simulink model "playback_data"  (R2015a)
settings: Solver=FixedStepDiscrete  SolverMode=SingleTasking  StartTime=76  StopTime=110  FixedStep=sample_time  RelTol=1e-3
undefined symbols (not defined in the file): A1_notch_f1, A2_notch_f1, A_kalman_swing_load, A_kalman_transverse, A_kalman_vertical, A_lpf_accelerometer, A_lpf_dtau, A_lpf_fourbar_angles, A_lpf_imu, A_lpf_lateral_angle, B1_lpf_accelerometer, B1_lpf_dtau, B1_lpf_fourbar_angles, B1_lpf_imu, B1_lpf_lateral_angle, B1_notch_f1, B2_lpf_accelerometer, B2_lpf_dtau, B2_lpf_fourbar_angles, B2_lpf_imu, B2_lpf_lateral_angle, B2_notch_f1, B_dx_versus_x0, B_kalman_swing_load, B_kalman_transverse, B_kalman_vertical, backwards_K_sag_of_t, backwards_P_sag_of_t, C_kalman_swing_load, C_kalman_transverse, C_kalman_vertical, com_leg_motor, com_torso, contact_threshold, control_start_time, d_ankle_to_foot, d_vertical_com, desired_com_forward_velocity, desired_com_lateral_velocity, desired_initial_leg_roll_left, desired_initial_leg_roll_right, desired_stance_beta2, desired_standing_torso_pitch, desired_standing_torso_roll, desired_standing_z, desired_torso_pitch, desired_torso_roll, Discrete, enable_bouncing, fcut_contact, fdesignblkfcn, forward_dx_of_dxstar, forward_x_of_dxstar, g, gcbh, HIP_MTR_MAX_CONT_TORQUE, HIP_MTR_MAX_TORQUE, i_leg_motor, i_robot, i_torso ... (+78)
libraries: simulink x65, dsparch4 x18, ctrlSharedLib x14, dspfdesign x4
(part 6 of 13)

== system playback_data/Control1/Actuator Control with Torque SEA commands/Timers ==
  Start [1/0] x4 : Inport
  Time [s] : Inport  Port=2
  Demux : Demux
  Mux : Mux
  Sum{8..11} (4 alike) : Sum  Inputs=|-+
  Time on Contact : Subsystem
  Time on Contact1 : Subsystem
  Time on Contact2 : Subsystem
  Time on Contact3 : Subsystem
  Timer [s] x4 : Outport
  wires:
  Sum10/1 -> Mux/3
  Sum11/1 -> Mux/4
  Demux/1 -> Time on Contact/Trigger
  Demux/4 -> Time on Contact3/Trigger
  Demux/3 -> Time on Contact2/Trigger
  Time on Contact3/1(out) -> Sum11/1
  Sum9/1 -> Mux/2
  Start [1/0] x4/1 -> Demux/1
  Sum8/1 -> Mux/1
  Time on Contact1/1(out) -> Sum9/1
  Demux/2 -> Time on Contact1/Trigger
  Time [s]/1 -> Time on Contact3/1(in), Time on Contact2/1(in), Time on Contact1/1(in), Time on Contact/1(in), Sum8/2, Sum9/2, Sum11/2, Sum10/2
  Mux/1 -> Timer [s] x4/1
  Time on Contact2/1(out) -> Sum10/1
  Time on Contact/1(out) -> Sum8/1

== system playback_data/Control1/Behavior Control/At Least One Stance Detected ==
  Enable : EnablePort  StatesWhenEnabling=reset
  Constant : Constant
  Stance? : Outport  InitialOutput=[0]
  wires:
  Constant/1 -> Stance?/1

== system playback_data/Control1/Behavior Control/Compute Forces1 ==
  XYZ Acceleration : Inport
  Constant5 : Constant  Value=g
  Demux : Demux  Outputs=3
  Gain4 : Gain  Gain=m_total_real
  Mux : Mux  Inputs=3
  Sum8 : Sum  Inputs=|++
  XYZ Force : Outport
  wires:
  Demux/1 -> Mux/1
  Demux/2 -> Mux/2
  Demux/3 -> Sum8/1
  Sum8/1 -> Mux/3
  Mux/1 -> Gain4/1
  Gain4/1 -> XYZ Force/1
  XYZ Acceleration/1 -> Demux/1
  Constant5/1 -> Sum8/2

== system playback_data/Control1/Behavior Control/Contact State Machine ==
  Contact Factor [body weight] : Inport
  "[Z dZ] [m m/s]" : Inport  Port=2
  ddZ [m/s^2] : Inport  Port=3
  Contact State : Scope
      settings: YMin=0.86  YMax=0.97  SaveName=ScopeData36  SampleInput=on
  Detect Fall Nonpositive : simulink/Logic and Bit Operations/Detect Fall Nonpositive  vinit=1  InputProcessing=Inherited  OutDataTypeStr=boolean
  Mux25 : Mux  Inputs=5
  Selector : Selector  InputPortWidth=2  Indices=[2]
  State Machine : State Transition Table  TreatAsAtomicUnit=on
  Unit Delay5 : UnitDelay  SampleTime=-1
  Unit Delay6 : UnitDelay  SampleTime=sample_time
  Unit Delay7 : UnitDelay  InitialCondition=1  SampleTime=sample_time
  flight [1/0] : Outport
  Exiting Stance [1/0] : Outport  Port=2
  wires:
  Detect Fall Nonpositive/1 -> Exiting Stance [1/0]/1
  Unit Delay7/1 -> flight [1/0]/1
  Unit Delay6/1 -> Detect Fall Nonpositive/1
  State Machine/4(" Takeoff") -> Unit Delay6/1, Mux25/4
  Selector/1 -> State Machine/1(z_velocity), Unit Delay5/1
  Contact Factor [body weight]/1 -> State Machine/3(vertical_grf)
  Unit Delay5/1 -> State Machine/2(previous_z_velocity)
  State Machine/5(" Flight") -> Mux25/5, Unit Delay7/1
  Mux25/1 -> Contact State/1
  State Machine/3(" Unloading") -> Mux25/3
  State Machine/2(" LockedContact") -> Mux25/2
  State Machine/1(" TouchDown") -> Mux25/1
  "[Z dZ] [m m/s]"/1 -> Selector/1
  ddZ [m/s^2]/1 -> State Machine/4(vertical_acceleration)

== system playback_data/Control1/Behavior Control/Estimate Angular Accelerations2 ==
  Angular Velocities [rad/s] x3 : Inport
  Enabled : Inport  Port=2
  Detect Change : simulink/Logic and Bit Operations/Detect Change  vinit=0  InputProcessing=Inherited  OutDataTypeStr=boolean
  Difference : simulink/Discrete/Difference  ICPrevInput=0.0  InputProcessing=Inherited  OutMin=[]  OutMax=[]  OutDataType=fixdt(1, 16)  OutScaling=2^-10  DoSatur=off
  Gain : Gain  Gain=1/sample_time
  IMU Two Pole Filter1 : DiscreteTransferFcn  Numerator=[A_lpf_imu 0 0]  Denominator=[1 B1_lpf_imu B2_lpf_imu]  SampleTime=sample_time
  Logical Operator5 : Logic  Operator=NOT  AllPortsSameDT=off  OutDataTypeStr=boolean
  Product : Product
  Angular Accelerations [rad/s^2] x3 : Outport
  wires:
  Enabled/1 -> Detect Change/1
  Logical Operator5/1 -> Product/2
  Product/1 -> IMU Two Pole Filter1/1
  Angular Velocities [rad/s] x3/1 -> Difference/1
  Gain/1 -> Product/1
  Difference/1 -> Gain/1
  Detect Change/1 -> Logical Operator5/1
  IMU Two Pole Filter1/1 -> Angular Accelerations [rad/s^2] x3/1

== system playback_data/Control1/Behavior Control/Estimate Angular Accelerations3 ==
  Angular Velocities [rad/s] x2 : Inport
  Enabled : Inport  Port=2
  Detect Change : simulink/Logic and Bit Operations/Detect Change  vinit=0  InputProcessing=Inherited  OutDataTypeStr=boolean
  Difference : simulink/Discrete/Difference  ICPrevInput=0.0  InputProcessing=Inherited  OutMin=[]  OutMax=[]  OutDataType=fixdt(1, 16)  OutScaling=2^-10  DoSatur=off
  Gain : Gain  Gain=1/sample_time
  Lateral Angle Two Pole Filter1 : DiscreteTransferFcn  Numerator=[A_lpf_lateral_angle 0 0]  Denominator=[1 B1_lpf_lateral_angle B2_lpf_lateral_angle]  SampleTime=sample_time
  Logical Operator5 : Logic  Operator=NOT  AllPortsSameDT=off  OutDataTypeStr=boolean
  Product : Product
  Angular Accelerations [rad/s^2] x2 : Outport
  wires:
  Detect Change/1 -> Logical Operator5/1
  Difference/1 -> Gain/1
  Gain/1 -> Product/1
  Angular Velocities [rad/s] x2/1 -> Difference/1
  Product/1 -> Lateral Angle Two Pole Filter1/1
  Logical Operator5/1 -> Product/2
  Enabled/1 -> Detect Change/1
  Lateral Angle Two Pole Filter1/1 -> Angular Accelerations [rad/s^2] x2/1

== system playback_data/Control1/Behavior Control/Exited Stance ==
  Enable : EnablePort  StatesWhenEnabling=reset
  Constant : Constant
  Takeoff? : Outport  InitialOutput=[0]
  wires:
  Constant/1 -> Takeoff?/1

== system playback_data/Control1/Behavior Control/Force Estimation ==
  Right/Left Primary : Inport
  Flight [1/0] : Inport  Port=2
  q : Inport  Port=3
  Torso Roll [rad rad/s] : Inport  Port=4
  Torso Pitch [rad rad/s] : Inport  Port=5
  Torso Yaw [rad rad/s] : Inport  Port=6
  Primary Leg Length [m m/s] : Inport  Port=7
  Primary Leg Angle [rad rad/s] : Inport  Port=8
  Primary Leg Roll [rad rad/s] : Inport  Port=9
  Secondary Leg Roll [rad rad/s] : Inport  Port=10
  Leg Width Right/Left [m m] : Inport  Port=11
  Leg Length Right/Left [m m] : Inport  Port=12
  Primary Lateral Torque [Nm] : Inport  Port=13
  Secondary Lateral Torque [Nm] : Inport  Port=14
  3D Forward Dynamics yawed : MATLAB Function  TreatAsAtomicUnit=on
  Constant : Constant  Value=m_total_real*g
  Demux : Demux  Outputs=2
  Divide : Product  Inputs=*/
  Lateral Motor Saturation : Saturate  UpperLimit=HIP_MTR_MAX_TORQUE  LowerLimit=-HIP_MTR_MAX_TORQUE
      settings: AttributesFormatString=Top: %<UpperLimit>\nBottom: %<LowerLimit>
  Lateral Motor Saturation1 : Saturate  UpperLimit=HIP_MTR_MAX_TORQUE  LowerLimit=-HIP_MTR_MAX_TORQUE
      settings: AttributesFormatString=Top: %<UpperLimit>\nBottom: %<LowerLimit>
  Leg Force Measurements : Subsystem
  Leg Plane GRF : Subsystem
  Logical Operator : Logic  Operator=NOT  AllPortsSameDT=off  OutDataTypeStr=boolean
  Mux : Mux  Inputs=2
  Mux1 : Mux  Inputs=2
  Product : Product
  Product2 : Product
  Product3 : Product
  Selector1 : Selector  InputPortWidth=2  Indices=[1]
  Selector2 : Selector  InputPortWidth=2  Indices=[1]
  Sum : Sum  Inputs=+|+
  Switch1 : Switch  Criteria=u2 ~= 0
  Switch2 : Switch  Criteria=u2 ~= 0
  Switch3 : Switch  Criteria=u2 ~= 0
  two_pole_filter : DiscreteTransferFcn  Numerator=[(1-2*exp(-fcut_contact*sample_time)+exp(-2*fcut_contact*sample_time)) 0 0]  Denominator=[1 (-2*exp(-fcut_contact*sample_time)) (exp(-2*fcut_contact*sample_time))]  SampleTime=sample_time
  Leg Plane Force for Contact Detection [body weight] : Outport
  Right GRF [X Y Z] [N N N] : Outport  Port=2
  Left GRF [X Y Z] [N N N] : Outport  Port=3
  GRF XYZ estimates [N N N] : Outport  Port=4  OutputWhenDisabled=reset  InitialOutput=[0 0 0 0 0 0]
  Torso Roll Acceleration [rad/s^2] : Outport  Port=5  OutputWhenDisabled=reset  InitialOutput=[0 0 0 0 0 0]
  wires:
  Divide/1 -> Leg Plane Force for Contact Detection [body weight]/1
  Leg Width Right/Left [m m]/1 -> Leg Force Measurements/2(Leg Width Right/Left [m m])
  q/1 -> Leg Force Measurements/1(q)
  two_pole_filter/1 -> Divide/1
  Constant/1 -> Divide/2
  [RightLeft] -> 3D Forward Dynamics yawed/1(right_or_left), Switch2/2, Switch1/2
  Leg Length Right/Left [m m]/1 -> Leg Force Measurements/3(Leg Length Right/Left [m m])
  3D Forward Dynamics yawed/1(R_GRF) -> Product2/2
  3D Forward Dynamics yawed/2(L_GRF) -> Product3/1
  3D Forward Dynamics yawed/3(ddroll) -> Product/1
  Leg Force Measurements/3(Right Leg Axial Force [N]) -> Mux/1, Switch1/1
  Leg Force Measurements/4(Left Leg Axial Force [N]) -> Switch1/3, Mux/2
  Switch1/1 -> 3D Forward Dynamics yawed/10(primary_leg_force)
  [TorsoPitch] -> 3D Forward Dynamics yawed/3(torso_pitch)
  Torso Roll [rad rad/s]/1 -> 3D Forward Dynamics yawed/2(torso_roll)
  Torso Yaw [rad rad/s]/1 -> 3D Forward Dynamics yawed/4(torso_yaw)
  Primary Leg Length [m m/s]/1 -> 3D Forward Dynamics yawed/6(primary_leg_length)
  [LegAngle] -> 3D Forward Dynamics yawed/5(primary_sagittal_leg_angle)
  Flight [1/0]/1 -> Logical Operator/1
  [Stance] -> Product/2
  Product/1 -> Torso Roll Acceleration [rad/s^2]/1
  Switch3/1 -> two_pole_filter/1
  Logical Operator/1 -> [Stance]
  Product3/1 -> Left GRF [X Y Z] [N N N]/1, Sum/2
  Product2/1 -> Right GRF [X Y Z] [N N N]/1, Sum/1
  [Stance] -> Product3/2
  [Stance] -> Product2/1
  Primary Leg Roll [rad rad/s]/1 -> 3D Forward Dynamics yawed/7(primary_leg_roll)
  Secondary Leg Roll [rad rad/s]/1 -> 3D Forward Dynamics yawed/8(secondary_leg_roll)
  Switch2/1 -> 3D Forward Dynamics yawed/9(primary_leg_torque)
  Leg Force Measurements/1(Right Leg Torque [Nm]) -> Switch2/1
  Leg Force Measurements/2(Left Leg Torque [Nm]) -> Switch2/3
  Sum/1 -> GRF XYZ estimates [N N N]/1
  Mux1/1 -> Leg Plane GRF/2(Orthogonal Force [N])
  Mux/1 -> Leg Plane GRF/1(Axial Force [N])
  Leg Force Measurements/5(Right Leg Orthogonal Force [N]) -> Mux1/1
  Leg Force Measurements/6(Left Leg Orthogonal Force [N]) -> Mux1/2
  Right/Left Primary/1 -> [RightLeft]
  [RightLeft] -> Switch3/2
  Leg Plane GRF/1(Vertical Force [N]) -> Demux/1
  Demux/1 -> Switch3/1
  Demux/2 -> Switch3/3
  Primary Leg Angle [rad rad/s]/1 -> [LegAngle]
  Torso Pitch [rad rad/s]/1 -> [TorsoPitch]
  [LegAngle] -> Selector1/1
  Selector1/1 -> Leg Plane GRF/4(Leg Angle [rad])
  [TorsoPitch] -> Selector2/1
  Selector2/1 -> Leg Plane GRF/3(Torso Pitch [rad])
  Primary Lateral Torque [Nm]/1 -> Lateral Motor Saturation/1
  Secondary Lateral Torque [Nm]/1 -> Lateral Motor Saturation1/1
  Lateral Motor Saturation/1 -> 3D Forward Dynamics yawed/11(primary_lateral_torque)
  Lateral Motor Saturation1/1 -> 3D Forward Dynamics yawed/12(secondary_lateral_torque)

== system playback_data/Control1/Behavior Control/L Leg Calculator ==
  Front [rad rad/s] : Inport
  Back [rad rad/s] : Inport  Port=2
  Constant : Constant  Value=d_ankle_to_foot-0.01
  Demux1 : Demux  Outputs=2
  Gain1 : Gain  Gain=2*l_seg
  Gain2 : Gain  Gain=l_seg
  Gain3 : Gain  Gain=-1
  Gain4 : Gain  Gain=0.5
  Gain5 : Gain  Gain=0.5
  Gain6 : Gain  Gain=2
  Mux1 : Mux  Inputs=2
  Product : Product  RndMeth=Zero
  Sum : Sum  Inputs=++|
  Sum4 : Sum  Inputs=+|+
  Sum5 : Sum  Inputs=+|-
  Trigonometric Function : Trigonometry  Operator=cos
  Trigonometric Function1 : Trigonometry
  "Leg Length [m m/s] " : Outport
  Leg Angle [rad rad/s] : Outport  Port=2
  Leg Splay [rad rad/s] : Outport  Port=3
  w [m] : Outport  Port=4
  wires:
  Sum/1 -> Mux1/1
  Constant/1 -> Sum/1
  Sum4/1 -> Gain5/1
  Mux1/1 -> "Leg Length [m m/s] "/1
  Sum5/1 -> Demux1/1, Leg Splay [rad rad/s]/1
  Gain2/1 -> Gain6/1, Product/1
  Demux1/1 -> Gain4/1
  Gain3/1 -> Product/2
  Demux1/2 -> Gain3/1
  Back [rad rad/s]/1 -> Sum5/1, Sum4/1
  Front [rad rad/s]/1 -> Sum4/2, Sum5/2
  Product/1 -> Mux1/2
  Trigonometric Function1/1 -> Gain2/1
  Gain1/1 -> Sum/2
  Trigonometric Function/1 -> Gain1/1
  Gain4/1 -> Trigonometric Function/1, Trigonometric Function1/1
  Gain6/1 -> w [m]/1
  Gain5/1 -> Leg Angle [rad rad/s]/1

== system playback_data/Control1/Behavior Control/Primary Secondary Leg Swap ==
  note: q Order:
      |
      | backJointR
      | backGearR
      | frontJointR
      | frontGearR
      |
      | backJointL
      | backGearL
      | frontJointL
      | frontGearL
      |
      | latR
      | latL
      |
      | boomRoll
      | boomYaw
      | boomPitch
  Exiting Stance [1/0] : Inport
  R Leg Angle [rad rad/s] : Inport  Port=2
  R Leg Length [m m/s] : Inport  Port=3
  R Leg w [m] : Inport  Port=4
  R Back Joint [rad rad/s] : Inport  Port=5
  R Back Gear [rad rad/s] : Inport  Port=6
  R Front Joint [rad rad/s] : Inport  Port=7
  R Front Gear [rad rad/s] : Inport  Port=8
  L Leg Angle [rad rad/s] : Inport  Port=9
  L Leg Length [m m/s] : Inport  Port=10
  L Leg w [m] : Inport  Port=11
  L Back Joint [rad rad/s] : Inport  Port=12
  L Back Gear [rad rad/s] : Inport  Port=13
  L Front Joint [rad rad/s] : Inport  Port=14
  L Front Gear [rad rad/s] : Inport  Port=15
  Primary Back/Front SEA Torque [Nm Nm] : Inport  Port=16
  Secondary Back/Front SEA Torque [Nm Nm] : Inport  Port=17
  "Right Leg Roll [rad, rad/s]" : Inport  Port=18
  "Left Leg Roll [rad, rad/s]" : Inport  Port=19
  Primary Lateral Torque [Nm] : Inport  Port=20
  Secondary Lateral Torque [Nm] : Inport  Port=21
  Primary Front/Back Velocity [rad/s rad/s] : Inport  Port=22
  Secondary Front/Back Velocity [rad/s rad/s] : Inport  Port=23
  Bus Creator : BusCreator  Inputs=22
  Bus Creator1 : BusCreator  Inputs=22
  Bus Selector : BusSelector  OutputSignals=signal1,signal2,signal3,signal4,signal5,signal6,signal7,signal8,signal9,signal10,signal11,signal12,signal13,signal14,signal15,signal16,signal17,signal18,signal19,signal20,signal21,signal22
  Manual Switch : ManualSwitch
  Select Leg : Constant  Value=initial_leg_selection  OutDataTypeStr=boolean
  Switch6 : Switch  Criteria=u2 ~= 0  OutDataTypeStr=Inherit: Inherit via back propagation  ZeroCross=off
  ToggleRightLeftLeg : MATLAB Function  TreatAsAtomicUnit=on
      settings: MinAlgLoopOccurrences=on
  Unit Delay : UnitDelay  InitialCondition=initial_leg_selection  SampleTime=sample_time
  Right/Left Primary [1/0] : Outport
  Primary Leg Angle [rad rad/s] : Outport  Port=2
  Primary Leg Length [m m/s] : Outport  Port=3
  Primary Leg w [m] : Outport  Port=4
  Primary Back Joint [rad rad/s] : Outport  Port=5
  Primary Back Gear [rad rad/s] : Outport  Port=6
  Primary Front Joint [rad rad/s] : Outport  Port=7
  Primary Front Gear [rad rad/s] : Outport  Port=8
  Secondary Leg Angle [rad rad/s] : Outport  Port=9
  Secondary Leg Length [rad rad/s] : Outport  Port=10
  Secondary Leg w [m] : Outport  Port=11
  Secondary Back Joint [rad rad/s] : Outport  Port=12
  Secondary Back Gear [rad rad/s] : Outport  Port=13
  Secondary Front Joint [rad rad/s] : Outport  Port=14
  Secondary Front Gear [rad rad/s] : Outport  Port=15
  R Back/Front SEA Torque [Nm Nm] : Outport  Port=16
  L Back/Front SEA Torque [Nm Nm] : Outport  Port=17
  "Primary Leg Roll [rad, rad/s]" : Outport  Port=18
  "Secondary Leg Roll [rad, rad/s]" : Outport  Port=19
  Right Lateral Torque [Nm] : Outport  Port=20
  Left Lateral Torque [Nm] : Outport  Port=21
  Right Front/Back Velocity [rad/s rad/s] : Outport  Port=22
  Left Front/Back Velocity [rad/s rad/s] : Outport  Port=23
  wires:
  Unit Delay/1 -> ToggleRightLeftLeg/2(previous_right_left)
  Exiting Stance [1/0]/1 -> ToggleRightLeftLeg/1(toggle)
  ToggleRightLeftLeg/1(right_left) -> Unit Delay/1, Manual Switch/1
  Manual Switch/1 -> Right/Left Primary [1/0]/1, Switch6/2
  Select Leg/1 -> Manual Switch/2
  R Leg Angle [rad rad/s]/1 -> Bus Creator1/8, Bus Creator/1
  Bus Creator/1 -> Switch6/1
  Bus Creator1/1 -> Switch6/3
  Switch6/1 -> Bus Selector/1
  R Leg Length [m m/s]/1 -> Bus Creator1/9, Bus Creator/2
  R Leg w [m]/1 -> Bus Creator1/10, Bus Creator/3
  R Back Joint [rad rad/s]/1 -> Bus Creator1/11, Bus Creator/4
  R Front Joint [rad rad/s]/1 -> Bus Creator1/13, Bus Creator/6
  R Front Gear [rad rad/s]/1 -> Bus Creator1/14, Bus Creator/7
  L Leg Angle [rad rad/s]/1 -> Bus Creator/8, Bus Creator1/1
  L Leg Length [m m/s]/1 -> Bus Creator1/2, Bus Creator/9
  L Leg w [m]/1 -> Bus Creator1/3, Bus Creator/10
  L Back Joint [rad rad/s]/1 -> Bus Creator1/4, Bus Creator/11
  L Back Gear [rad rad/s]/1 -> Bus Creator1/5, Bus Creator/12
  L Front Joint [rad rad/s]/1 -> Bus Creator1/6, Bus Creator/13
  L Front Gear [rad rad/s]/1 -> Bus Creator1/7, Bus Creator/14
  Primary Back/Front SEA Torque [Nm Nm]/1 -> Bus Creator1/16, Bus Creator/15
  Secondary Back/Front SEA Torque [Nm Nm]/1 -> Bus Creator1/15, Bus Creator/16
  "Right Leg Roll [rad, rad/s]"/1 -> Bus Creator1/18, Bus Creator/17
  "Left Leg Roll [rad, rad/s]"/1 -> Bus Creator1/17, Bus Creator/18
  Primary Lateral Torque [Nm]/1 -> Bus Creator1/20, Bus Creator/19
  Secondary Lateral Torque [Nm]/1 -> Bus Creator1/19, Bus Creator/20
  R Back Gear [rad rad/s]/1 -> Bus Creator1/12, Bus Creator/5
  Bus Selector/1 -> Primary Leg Angle [rad rad/s]/1  "<signal1>"
  Bus Selector/2 -> Primary Leg Length [m m/s]/1  "<signal2>"
  Bus Selector/3 -> Primary Leg w [m]/1  "<signal3>"
  Bus Selector/4 -> Primary Back Joint [rad rad/s]/1  "<signal4>"
  Bus Selector/5 -> Primary Back Gear [rad rad/s]/1  "<signal5>"
  Bus Selector/6 -> Primary Front Joint [rad rad/s]/1  "<signal6>"
  Bus Selector/7 -> Primary Front Gear [rad rad/s]/1  "<signal7>"
  Bus Selector/8 -> Secondary Leg Angle [rad rad/s]/1  "<signal8>"
  Bus Selector/9 -> Secondary Leg Length [rad rad/s]/1  "<signal9>"
  Bus Selector/10 -> Secondary Leg w [m]/1  "<signal10>"
  Bus Selector/11 -> Secondary Back Joint [rad rad/s]/1  "<signal11>"
  Bus Selector/12 -> Secondary Back Gear [rad rad/s]/1  "<signal12>"
  Bus Selector/13 -> Secondary Front Joint [rad rad/s]/1  "<signal13>"
  Bus Selector/14 -> Secondary Front Gear [rad rad/s]/1  "<signal14>"
  Bus Selector/15 -> R Back/Front SEA Torque [Nm Nm]/1  "<signal15>"
  Bus Selector/16 -> L Back/Front SEA Torque [Nm Nm]/1  "<signal16>"
  Bus Selector/17 -> "Primary Leg Roll [rad, rad/s]"/1  "<signal17>"
  Bus Selector/18 -> "Secondary Leg Roll [rad, rad/s]"/1  "<signal18>"
  Bus Selector/19 -> Right Lateral Torque [Nm]/1  "<signal19>"
  Bus Selector/20 -> Left Lateral Torque [Nm]/1  "<signal20>"
  Primary Front/Back Velocity [rad/s rad/s]/1 -> Bus Creator1/22, Bus Creator/21
  Secondary Front/Back Velocity [rad/s rad/s]/1 -> Bus Creator1/21, Bus Creator/22
  Bus Selector/21 -> Right Front/Back Velocity [rad/s rad/s]/1  "<signal21>"
  Bus Selector/22 -> Left Front/Back Velocity [rad/s rad/s]/1  "<signal22>"

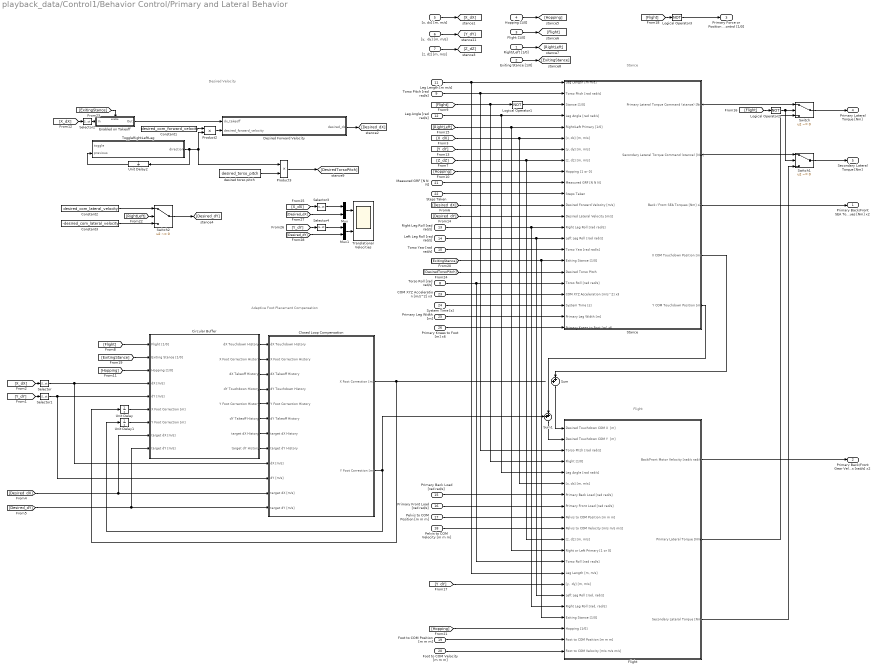
== system playback_data/Control1/Behavior Control/Primary and Lateral Behavior ==
  note: Stance
  note: Flight
  note: Adaptive Foot Placement Compensation
  note: Desired Velocity
  Right/Left [1/0] : Inport
  Exiting Stance [1/0] : Inport  Port=2
  Flight [1/0] : Inport  Port=3
  Hopping [1/0] : Inport  Port=4
  "[x, dx] [m, m/s]" : Inport  Port=5
  "[y,  dy] [m, m/s]" : Inport  Port=6
  "[z, dz] [m, m/s]" : Inport  Port=7
  Torso Roll [rad rad/s] : Inport  Port=8
  Torso Pitch [rad rad/s] : Inport  Port=9
  Torso Yaw [rad rad/s] : Inport  Port=10
  Leg Length [m m/s] : Inport  Port=11
  Leg Angle [rad rad/s] : Inport  Port=12
  Right Leg Roll [rad rad/s] : Inport  Port=13
  Left Leg Roll [rad rad/s] : Inport  Port=14
  Primary Back Load [rad rad/s] : Inport  Port=15
  Primary Front Load [rad rad/s] : Inport  Port=16
  Pelvis to COM Position [m m m] : Inport  Port=17
  Pelvis to COM Velocity [m m m] : Inport  Port=18
  Foot to COM Position [m m m] : Inport  Port=19
  Foot to COM Velocity [m m m] : Inport  Port=20
  Measured GRF [N N N] : Inport  Port=21
  Steps Taken : Inport  Port=22
  COM XYZ Acceleration [m/s^2] x3 : Inport  Port=23
  System Time [s] : Inport  Port=24
  Primary Leg Width [m] : Inport  Port=25
  Primary Knees to Foot [m] x6 : Inport  Port=26
  Circular Buffer : Subsystem
  Closed Loop Compensation : Subsystem
  Constant1 : Constant  Value=desired_com_forward_velocity
  Constant2 : Constant  Value=desired_com_lateral_velocity
  Constant3 : Constant  Value=-desired_com_lateral_velocity
  Desired Forward Velocity : MATLAB Function  TreatAsAtomicUnit=on
  Enabled on Takeoff : Subsystem  TreatAsAtomicUnit=on
  Flight : Subsystem
  Logical Operator1 : Logic  Operator=NOT  AllPortsSameDT=off  OutDataTypeStr=boolean
  Logical Operator2 : Logic  Operator=NOT  AllPortsSameDT=off  OutDataTypeStr=boolean
  Logical Operator3 : Logic  Operator=NOT  AllPortsSameDT=off  OutDataTypeStr=boolean
  Mux : Mux  Inputs=2
  Mux1 : Mux  Inputs=2
  Product2 : Product
  Product3 : Product
  Selector{,1..4} (5 alike) : Selector  InputPortWidth=2  Indices=[2]
  Stance : Subsystem
  Sum : Sum  Inputs=++|
  Sum1 : Sum  Inputs=++|
  Switch : Switch  Criteria=u2 ~= 0
  Switch1 : Switch  Criteria=u2 ~= 0
  Switch2 : Switch  Criteria=u2 ~= 0
  ToggleRightLeftLeg : MATLAB Function  TreatAsAtomicUnit=on
      settings: MinAlgLoopOccurrences=on
  Translational Velocities : Scope  NumInputPorts=2
      settings: YMin=-1000~-5  YMax=1000~5  SaveName=ScopeData2  SampleInput=on
  Unit Delay : UnitDelay  SampleTime=-1
  Unit Delay1 : UnitDelay  SampleTime=-1
  Unit Delay2 : UnitDelay  InitialCondition=1  SampleTime=sample_time
  desired torso pitch : Constant  Value=desired_torso_pitch
  Primary Back/Front SEA Torques [Nm] x2 : Outport
  Primary Back/Front Gear Velocities [rad/s] x2 : Outport  Port=2
  Primary Force or Position Control [1/0] : Outport  Port=3  OutDataTypeStr=boolean
  Primary Lateral Torque [Nm] : Outport  Port=4
  Secondary Lateral Torque [Nm] : Outport  Port=5
  wires:
  Leg Length [m m/s]/1 -> Stance/1(Leg Length [m m/s]), Flight/14("Leg Length [m, m/s]")
  Torso Pitch [rad rad/s]/1 -> Stance/2(Torso Pitch [rad rad/s]), Flight/3(Torso Pitch [rad rad/s])
  [Hopping] -> Stance/9(Hopping [1 or 0])
  [X_dX] -> Flight/6("[x, dx] [m, m/s]"), Stance/6("[x, dx] [m, m/s]")
  [RightLeft] -> Flight/12(Right or Left Primary [1 or 0]), Stance/5(Right/Left Primary [1/0])
  Primary Back Load [rad rad/s]/1 -> Flight/7(Primary Back Load [rad rad/s])
  Primary Front Load [rad rad/s]/1 -> Flight/8(Primary Front Load [rad rad/s])
  Leg Angle [rad rad/s]/1 -> Flight/5(Leg Angle [rad rad/s]), Stance/4(Leg Angle [rad rad/s])
  Flight/1(Back/Front Motor Velocity [rad/s rad/s]) -> Primary Back/Front Gear Velocities [rad/s] x2/1
  Logical Operator1/1 -> Stance/3(Stance [1/0])
  [Flight] -> Circular Buffer/1(Flight [1/0])
  Pelvis to COM Position [m m m]/1 -> Flight/9(Pelvis to COM Position [m m m])
  [Z_dZ] -> Stance/8("[z, dz] [m, m/s]"), Flight/11("[z, dz] [m, m/s]")
  Pelvis to COM Velocity [m m m]/1 -> Flight/10(Pelvis to COM Velocity [m/s m/s m/s])
  Torso Roll [rad rad/s]/1 -> Flight/13(Torso Roll [rad rad/s]), Stance/19(Torso Roll [rad rad/s])
  Measured GRF [N N N]/1 -> Stance/10(Measured GRF [N N N])
  Steps Taken/1 -> Stance/11(Steps Taken)
  [Y_dY] -> Flight/15("[y,  dy] [m, m/s]")
  Circular Buffer/1("dX Touchdown History ") -> Closed Loop Compensation/1(dX Touchdown History)
  Circular Buffer/2(X Foot Correction History) -> Closed Loop Compensation/2(X Foot Correction History)
  Circular Buffer/3(dX Takeoff History) -> Closed Loop Compensation/3(dX Takeoff History)
  Circular Buffer/4("dY Touchdown History ") -> Closed Loop Compensation/4(dY Touchdown History)
  Circular Buffer/5(Y Foot Correction History) -> Closed Loop Compensation/5(Y Foot Correction History)
  Circular Buffer/6(dY Takeoff History) -> Closed Loop Compensation/6(dY Takeoff History)
  Circular Buffer/8(target dY History) -> Closed Loop Compensation/8(target dY History)
  Circular Buffer/7(target dX History) -> Closed Loop Compensation/7(target dX History)
  [Desired_dX] -> Circular Buffer/8(target dX [m/s]), Closed Loop Compensation/11(target dX [m/s])
  [Desired_dY] -> Circular Buffer/9(target dY [m/s]), Closed Loop Compensation/12("target dY [m/s] ")
  Stance/4(X COM Touchdown Position [m]) -> Sum/2
  Sum/1 -> Flight/1(Desired Touchdown COM X  [m])
  Closed Loop Compensation/1(X Foot Correction [m]) -> Unit Delay/1
  Selector1/1 -> Circular Buffer/5(dY [m/s]), Closed Loop Compensation/10(dY [m/s])
  Selector/1 -> Circular Buffer/4(dX [m/s]), Closed Loop Compensation/9(dX [m/s])
  Unit Delay1/1 -> Circular Buffer/7(Y Foot Correction [m])
  Unit Delay/1 -> Circular Buffer/6(X Foot Correction [m])
  Closed Loop Compensation/2(Y Foot Correction [m]) -> Unit Delay1/1, Sum1/1
  "[x, dx] [m, m/s]"/1 -> [X_dX]
  "[z, dz] [m, m/s]"/1 -> [Z_dZ]
  "[y,  dy] [m, m/s]"/1 -> [Y_dY]
  [X_dX] -> Selector/1
  [Y_dY] -> Selector1/1
  [Desired_dX] -> Stance/12(Desired Forward Velocity [m/s])
  Flight [1/0]/1 -> [Flight]
  [Flight] -> Flight/4(Flight [1/0]), Logical Operator1/1
  Hopping [1/0]/1 -> [Hopping]
  Stance/5(Y COM Touchdown Position [m]) -> Sum1/2
  Sum1/1 -> Flight/2(Desired Touchdown COM Y  [m])
  Right Leg Roll [rad rad/s]/1 -> Flight/17("Right Leg Roll [rad, rad/s]"), Stance/14(Right Leg Roll [rad rad/s])
  Left Leg Roll [rad rad/s]/1 -> Flight/16("Left Leg Roll [rad, rad/s]"), Stance/15(Left Leg Roll [rad rad/s])
  [Y_dY] -> Stance/7("[y, dy] [m, m/s]")
  [Desired_dY] -> Stance/13(Desired Lateral Velocity [m/s])
  Right/Left [1/0]/1 -> [RightLeft]
  Logical Operator2/1 -> Switch1/2, Switch/2
  Flight/2(Primary Lateral Torque [Nm]) -> Switch/3
  Flight/3(Secondary Lateral Torque [Nm]) -> Switch1/3
  [Flight] -> Logical Operator2/1
  Switch/1 -> Primary Lateral Torque [Nm]/1
  Switch1/1 -> Secondary Lateral Torque [Nm]/1
  [Flight] -> Logical Operator3/1
  Logical Operator3/1 -> Primary Force or Position Control [1/0]/1
  Torso Yaw [rad rad/s]/1 -> Stance/16(Torso Yaw [rad rad/s])
  [Hopping] -> Circular Buffer/3(Hopping [1/0])
  [ExitingStance] -> Circular Buffer/2(Exiting Stance [1/0])
  Exiting Stance [1/0]/1 -> [ExitingStance]
  [ExitingStance] -> Flight/18(Exiting Stance [1/0]), Stance/17(Exiting Stance [1/0])
  [Hopping] -> Flight/19(Hopping [1/0])
  [X_dX] -> Selector2/1
  Switch2/1 -> [Desired_dY]
  Enabled on Takeoff/1(Out) -> Desired Forward Velocity/1(dx_takeoff)
  [RightLeft] -> Switch2/2
  Constant2/1 -> Switch2/1
  Constant3/1 -> Switch2/3
  [ExitingStance] -> Enabled on Takeoff/Enable
  Selector2/1 -> Enabled on Takeoff/1(In)
  Desired Forward Velocity/1(desired_dx) -> [Desired_dX]
  Product2/1 -> Desired Forward Velocity/2(desired_forward_velocity)
  ToggleRightLeftLeg/1(direction) -> Product2/2, Product3/1, Unit Delay2/1
  Unit Delay2/1 -> ToggleRightLeftLeg/2(previous)
  Constant1/1 -> Product2/1
  desired torso pitch/1 -> Product3/2
  Product3/1 -> [DesiredTorsoPitch]
  [DesiredTorsoPitch] -> Stance/18(Desired Torso Pitch)
  Foot to COM Position [m m m]/1 -> Flight/20(Foot to COM Position [m m m])
  Foot to COM Velocity [m m m]/1 -> Flight/21(Foot to COM Velocity [m/s m/s m/s])
  [X_dX] -> Selector3/1
  Selector3/1 -> Mux/1
  [Y_dY] -> Selector4/1
  Selector4/1 -> Mux1/1
  Mux/1 -> Translational Velocities/1
  Mux1/1 -> Translational Velocities/2
  [Desired_dY] -> Mux1/2
  [Desired_dX] -> Mux/2
  COM XYZ Acceleration [m/s^2] x3/1 -> Stance/20(COM XYZ Acceleration [m/s^2] x3)
  System Time [s]/1 -> Stance/21(System Time [s])
  Primary Leg Width [m]/1 -> Stance/22(Primary Leg Width [m])
  Stance/2(Secondary Lateral Torque Command (stance) [Nm]) -> Switch1/1
  Stance/3(Back / Front SEA Torques [Nm] x2) -> Primary Back/Front SEA Torques [Nm] x2/1
  Stance/1(Primary Lateral Torque Command (stance) [Nm]) -> Switch/1
  Primary Knees to Foot [m] x6/1 -> Stance/23(Primary Knees to Foot [m] x6)

== system playback_data/Control1/Behavior Control/R Leg Calculator ==
  Front [rad rad/s] : Inport
  Back [rad rad/s] : Inport  Port=2
  Constant : Constant  Value=d_ankle_to_foot-0.01
  Demux1 : Demux  Outputs=2
  Gain1 : Gain  Gain=2*l_seg
  Gain2 : Gain  Gain=l_seg
  Gain3 : Gain  Gain=-1
  Gain4 : Gain  Gain=0.5
  Gain5 : Gain  Gain=0.5
  Gain6 : Gain  Gain=2
  Mux1 : Mux  Inputs=2
  Product : Product  RndMeth=Zero
  Sum : Sum  Inputs=++|
  Sum4 : Sum  Inputs=+|+
  Sum5 : Sum  Inputs=+|-
  Trigonometric Function : Trigonometry  Operator=cos
  Trigonometric Function1 : Trigonometry
  "Leg Length [m m/s] " : Outport
  Leg Angle [rad rad/s] : Outport  Port=2
  Leg Splay [rad rad/s] : Outport  Port=3
  w [m] : Outport  Port=4
  wires:
  Constant/1 -> Sum/1
  Sum/1 -> Mux1/1
  Gain6/1 -> w [m]/1
  Gain4/1 -> Trigonometric Function1/1, Trigonometric Function/1
  Trigonometric Function/1 -> Gain1/1
  Gain1/1 -> Sum/2
  Trigonometric Function1/1 -> Gain2/1
  Product/1 -> Mux1/2
  Front [rad rad/s]/1 -> Sum5/2, Sum4/2
  Back [rad rad/s]/1 -> Sum4/1, Sum5/1
  Demux1/2 -> Gain3/1
  Gain3/1 -> Product/2
  Demux1/1 -> Gain4/1
  Gain2/1 -> Product/1, Gain6/1
  Sum5/1 -> Leg Splay [rad rad/s]/1, Demux1/1
  Mux1/1 -> "Leg Length [m m/s] "/1
  Sum4/1 -> Gain5/1
  Gain5/1 -> Leg Angle [rad rad/s]/1

== system playback_data/Control1/Behavior Control/Secondary Leg Behavior ==
  note: Mirror the primary
      | leg motion
  note: Position control the
      | individual four bar segments
  note: Convert to
      | four-bar angles
  Secondary Back Load [rad rad/s] : Inport
  Secondary Front Load [rad rad/s] : Inport  Port=2
  Torso Pitch [rad rad/s] : Inport  Port=3
  Primary Leg Angle [rad rad/s] : Inport  Port=4
  Primary Leg Length [m m/s] : Inport  Port=5
  Avoid Hitting Mechanical Limits : MATLAB Function  TreatAsAtomicUnit=on
  Back/Front PD : Subsystem
  Constant4 : Constant  Value=0
  Demux{1..3,5} (4 alike) : Demux  Outputs=2
  Demux6 : Demux  Outputs=6
  Fcn2 : Fcn  Expr=2*pi-u(1)
  Lowpass Filter (Swing) : Subsystem  DialogController=fdesignblkfcn  InitFcn=fdesignblkfcn(gcbh, {'InitFcn'});  mask(Lowpass Filter){}
      mask help: Design a lowpass filter
      settings: CopyFcn=fdesignblkfcn(gcbh, {'CopyFcn'});
      mask Help: helpview(mapfilelocation('dsp'), 'dsplowpassfilter');
      mask Display: disp('Lowpass')
  Mirrored Leg Length Target : MATLAB Function  TreatAsAtomicUnit=on
  Mux{1..4,7,11} (6 alike) : Mux  Inputs=2
  Mux5 : Mux  Inputs=3
  Mux6 : Mux  Inputs=3
  Sum : Sum  Inputs=++|
  Terminator : Terminator
  Virtual Leg to Four Bar : MATLAB Function  TreatAsAtomicUnit=on
  k_virtual1 : Gain  Gain=2
  k_virtual6 : Gain  Gain=-1
  Secondary Back/Front Motor Torque [Nm Nm] : Outport
  wires:
  Demux5/1 -> Fcn2/1
  Mirrored Leg Length Target/2(dl_leg) -> Mux5/2
  Mirrored Leg Length Target/3(ddl_leg) -> Mux5/3
  Mirrored Leg Length Target/1(l_leg) -> Mux5/1
  Constant4/1 -> Mux6/3
  k_virtual6/1 -> Mux6/2
  Fcn2/1 -> Mux6/1
  Mux7/1 -> Demux6/1
  Virtual Leg to Four Bar/1(back) -> Avoid Hitting Mechanical Limits/1(back_desired)
  Virtual Leg to Four Bar/2(dback) -> Avoid Hitting Mechanical Limits/2(dback_desired)
  Virtual Leg to Four Bar/3(ddback) -> Avoid Hitting Mechanical Limits/3(ddback_desired)
  Virtual Leg to Four Bar/4(front) -> Avoid Hitting Mechanical Limits/4(front_desired)
  Virtual Leg to Four Bar/5(dfront) -> Avoid Hitting Mechanical Limits/5(dfront_desired)
  Virtual Leg to Four Bar/6(ddfront) -> Avoid Hitting Mechanical Limits/6(ddfront_desired)
  Demux6/1 -> Virtual Leg to Four Bar/1(l_leg)
  Demux6/2 -> Virtual Leg to Four Bar/2(dl_leg)
  Demux6/3 -> Virtual Leg to Four Bar/3(ddl_leg)
  Demux6/4 -> Virtual Leg to Four Bar/4(phi)
  Demux6/5 -> Virtual Leg to Four Bar/5(dphi)
  Demux6/6 -> Virtual Leg to Four Bar/6(ddphi)
  Mux11/1 -> Back/Front PD/4(Measured Velocity [rad/s] [back front])
  Demux2/2 -> Mux11/2
  Mux4/1 -> Back/Front PD/3(Measured Position [rad] [back front])
  Mux1/1 -> Back/Front PD/1(Desired Position [rad] [back front])
  Demux3/2 -> Mux11/1
  Demux3/1 -> Mux4/1
  Avoid Hitting Mechanical Limits/2(front_cmd) -> Mux1/2
  Avoid Hitting Mechanical Limits/1(back_cmd) -> Mux1/1
  Demux2/1 -> Mux4/2
  Secondary Front Load [rad rad/s]/1 -> Demux2/1
  Secondary Back Load [rad rad/s]/1 -> Demux3/1
  Avoid Hitting Mechanical Limits/3(dback_cmd) -> Mux2/1
  Avoid Hitting Mechanical Limits/4(dfront_cmd) -> Mux2/2
  Avoid Hitting Mechanical Limits/5(ddback_cmd) -> Mux3/1
  Avoid Hitting Mechanical Limits/6(ddfront_cmd) -> Mux3/2
  Mux2/1 -> Back/Front PD/2(Desired Velocity [rad/s] [back front])
  Primary Leg Angle [rad rad/s]/1 -> Sum/2
  Demux1/1 -> Mirrored Leg Length Target/1(primary_l_leg)
  Demux1/2 -> Mirrored Leg Length Target/2(primary_dl_leg)
  Primary Leg Length [m m/s]/1 -> Demux1/1
  Sum/1 -> Demux5/1
  Torso Pitch [rad rad/s]/1 -> k_virtual1/1
  k_virtual1/1 -> Sum/1
  Mux5/1 -> Mux7/1
  Mux3/1 -> Terminator/1
  Demux5/2 -> k_virtual6/1
  Mux6/1 -> Mux7/2
  Back/Front PD/1(Commanded Velocity [rad/s] [back front]) -> Lowpass Filter (Swing)/1(In)
  Lowpass Filter (Swing)/1(Out) -> Secondary Back/Front Motor Torque [Nm Nm]/1

== system playback_data/Control1/Behavior Control/State Estimation ==
  Right or Left [1/0] : Inport
  Torso Roll [rad rad/s] : Inport  Port=2
  Torso Pitch [rad rad/s] : Inport  Port=3
  Torso Yaw [rad rad/s] : Inport  Port=4
  Left Leg Sagittal Angle [rad rad/s] : Inport  Port=5
  Left Leg Roll [rad rad/s] : Inport  Port=6
  Left Leg Length [m m/s] : Inport  Port=7
  Right Leg Sagittal Angle [rad rad/s] : Inport  Port=8
  Right Leg Roll [rad rad/s] : Inport  Port=9
  Right Leg Length [m m/s] : Inport  Port=10
  Enable Kalman Filtering [1/0] : Inport  Port=11
  Right GRF [X Y Z] [N N N] : Inport  Port=12
  Left GRF [X Y Z] [N N N] : Inport  Port=13
  " Acceleration Measurement [m/s^2] x3" : Inport  Port=14
  Flight [1/0] : Inport  Port=15
  Right Back [rad rad/s] : Inport  Port=16
  Left Back [rad rad/s] : Inport  Port=17
  Right Front [rad rad/s] : Inport  Port=18
  Left Front [rad rad/s] : Inport  Port=19
  ComputeKneePositions : MATLAB Function  TreatAsAtomicUnit=on
  Demux{,1..7} (8 alike) : Demux  Outputs=3
  Demux11 : Demux  Outputs=2
  Demux8 : Demux  Outputs=2
  Detect Decrease : simulink/Logic and Bit Operations/Detect Decrease  vinit=0.0  InputProcessing=Inherited  OutDataTypeStr=boolean
  Discrete Derivative : simulink/Discrete/Discrete Derivative  gainval=1.0  ICPrevScaledInput=0.0  InputProcessing=Inherited  OutMin=[]  OutMax=[]  OutDataType=fixdt(1, 16)  OutScaling=2^-10  DoSatur=off
  Discrete Derivative1 : simulink/Discrete/Discrete Derivative  gainval=1.0  ICPrevScaledInput=0.0  InputProcessing=Inherited  OutMin=[]  OutMax=[]  OutDataType=fixdt(1, 16)  OutScaling=2^-10  DoSatur=off
  Discrete-Time Integrator : DiscreteIntegrator  InitialConditionSetting=State (most efficient)  SampleTime=-1
  Discrete-Time Integrator1 : DiscreteIntegrator  InitialConditionSetting=State (most efficient)  SampleTime=-1
  Kalman Filtering : Subsystem
  L Front Back Knee to Foot : Scope  NumInputPorts=2
      settings: YMin=-0.425~-0.5  YMax=-0.025~0.3  SaveName=ScopeData44  SampleInput=on
  Lowpass Filter : Subsystem  DialogController=fdesignblkfcn  InitFcn=fdesignblkfcn(gcbh, {'InitFcn'});  mask(Lowpass Filter){}
      mask help: Design a lowpass filter
      settings: CopyFcn=fdesignblkfcn(gcbh, {'CopyFcn'});
      mask Help: helpview(mapfilelocation('dsp'), 'dsplowpassfilter');
      mask Display: disp('Lowpass')
  Mux{,1,3,5,8..9,12..13} (8 alike) : Mux  Inputs=3
  Mux{2,4,6..7,10,14..20} (12 alike) : Mux  Inputs=2
  Mux11 : Mux
  PositionUsingRobotGeometry : MATLAB Function  TreatAsAtomicUnit=on
  Selector : Selector  InputPortWidth=3  Indices=[3]
  Selector1 : Selector  InputPortWidth=3  Indices=[3]
  Sum : Sum  Inputs=|++
  Switch : Switch  Criteria=u2 ~= 0
  Switch1 : Switch  Criteria=u2 ~= 0
  Switch2 : Switch  Criteria=u2 ~= 0
  Terminator6 : Terminator
  X Kalman Output : Scope  NumInputPorts=3
      settings: TimeRange=3.774467455621291  YMin=5.55112e-17~-0.075~-0.5  YMax=2.1~0.25~0.6  SaveName=ScopeData29  SampleInput=on
  Y Kalman Output : Scope  NumInputPorts=3
      settings: TimeRange=39.999  YMin=0.05~-0.7~-2  YMax=0.18~1.1~3.5  SaveName=ScopeData30  SampleInput=on
  Z Kalman Output : Scope  NumInputPorts=3
      settings: TimeRange=3.175000000000004  YMin=0~-0.04~-0.7  YMax=0.9~0.035~0.6  SaveName=ScopeData27  SampleInput=on
  "[ddx, ddy, ddz]" : Selector  InputPortWidth=9  Indices=[3 6 9]
  "[x dx]" : Selector  InputPortWidth=9  Indices=[1 2]
  "[y dy]" : Selector  InputPortWidth=9  Indices=[4 5]
  "[z dz]" : Selector  InputPortWidth=9  Indices=[7 8]
  body frame : Selector  InputPortWidth=9  Indices=[1 2 3]
  body frame1 : Selector  InputPortWidth=9  Indices=[1 2 3]
  body frame{2..5} (4 alike) : Selector  InputPortWidth=9  Indices=[4 5 6]
  body frame{6..9} (4 alike) : Selector  InputPortWidth=9  Indices=[7 8 9]
  "Horizontal COM [m, m/s]" : Outport
  "Lateral COM [m, m/s]" : Outport  Port=2
  "Vertical COM [m, m/s]" : Outport  Port=3
  Pelvis to COM Position [m m m] : Outport  Port=4
  Pelvis to COM Velocity [m/s m/s m/s] : Outport  Port=5
  Foot to COM Position [m m m] : Outport  Port=6
  Foot to COM Velocity [m/s m/s m/s] : Outport  Port=7
  COM Acceleration [m/s^2] x3 : Outport  Port=8
  Right Knees to Foot [m m m] x2 : Outport  Port=9
  Left Knees to Foot [m m m] x2 : Outport  Port=10
  COM Position World [m m m] : Outport  Port=11  PortDimensions=3
  COM Velocity World [m/s m/s m/s] : Outport  Port=12  PortDimensions=3
  wires:
  Discrete-Time Integrator1/1 -> Mux13/3
  Lowpass Filter/1(Out) -> Mux12/3
  Discrete Derivative/1 -> Lowpass Filter/1(In)
  Discrete-Time Integrator/1 -> Discrete-Time Integrator1/1, Mux11/3
  Demux5/3 -> Mux12/1, Discrete-Time Integrator/1
  Demux5/2 -> Mux11/1, Discrete Derivative/1
  Demux5/1 -> Mux13/1
  Demux4/3 -> Mux12/2
  Mux11/1 -> X Kalman Output/2
  Demux4/1 -> Discrete Derivative1/1, Mux13/2
  Demux4/2 -> Mux11/2
  Mux13/1 -> X Kalman Output/1
  Mux12/1 -> X Kalman Output/3
  Mux9/1 -> Mux3/2, Demux7/1, Kalman Filtering/9("Initial [y, dy, ddy] [m, m/s, m/s^2]")
  Mux8/1 -> Mux3/1, Demux5/1, Kalman Filtering/8("Initial [x, dx, ddx] [m, m/s, m/s^2]")
  "[ddx, ddy, ddz]"/1 -> COM Acceleration [m/s^2] x3/1
  Mux3/1 -> Switch/3
  Demux2/2 -> Mux9/3
  Demux2/1 -> Mux8/3
  Demux2/3 -> Mux/3
  " Acceleration Measurement [m/s^2] x3"/1 -> Demux2/1, Kalman Filtering/11(COM XYZ Acceleration [m/s^2] x3)
  PositionUsingRobotGeometry/5(horizontal_com_position) -> Mux8/1
  Left Leg Sagittal Angle [rad rad/s]/1 -> PositionUsingRobotGeometry/5(left_leg_sagittal_angle), ComputeKneePositions/4(left_leg_sagittal_angle)
  Left Leg Roll [rad rad/s]/1 -> PositionUsingRobotGeometry/6(left_leg_lateral_angle), ComputeKneePositions/5(left_leg_lateral_angle)
  Left Leg Length [m m/s]/1 -> PositionUsingRobotGeometry/7(left_leg_length), ComputeKneePositions/6(left_leg_length)
  Right Leg Sagittal Angle [rad rad/s]/1 -> PositionUsingRobotGeometry/8(right_leg_sagittal_angle), ComputeKneePositions/7(right_leg_sagittal_angle)
  Right Leg Roll [rad rad/s]/1 -> ComputeKneePositions/8(right_leg_lateral_angle), PositionUsingRobotGeometry/9(right_leg_lateral_angle)
  Right Leg Length [m m/s]/1 -> ComputeKneePositions/9(right_leg_length), PositionUsingRobotGeometry/10(right_leg_length)
  Right or Left [1/0]/1 -> [RightLeftPrimary], PositionUsingRobotGeometry/1(right_left)
  Torso Roll [rad rad/s]/1 -> PositionUsingRobotGeometry/2(roll), ComputeKneePositions/1(roll)
  Torso Yaw [rad rad/s]/1 -> PositionUsingRobotGeometry/4(yaw), ComputeKneePositions/3(yaw)
  Torso Pitch [rad rad/s]/1 -> PositionUsingRobotGeometry/3(pitch), ComputeKneePositions/2(pitch)
  Mux5/1 -> Switch/1
  Selector/1 -> Kalman Filtering/6(Right Vertical GRF [N])
  Selector1/1 -> Kalman Filtering/7(Left Vertical GRF [N])
  Left GRF [X Y Z] [N N N]/1 -> Selector1/1, Sum/2
  Right GRF [X Y Z] [N N N]/1 -> Selector/1, Sum/1
  Sum/1 -> Demux/1
  Enable Kalman Filtering [1/0]/1 -> Kalman Filtering/Enable, [EnableKalmanFiltering]
  Demux/1 -> Kalman Filtering/3(GRFx [N])
  Mux1/1 -> Terminator6/1
  PositionUsingRobotGeometry/12(dcom_pelvis) -> body frame1/1
  PositionUsingRobotGeometry/11(com_pelvis) -> body frame/1
  "[x dx]"/1 -> "Horizontal COM [m, m/s]"/1
  body frame/1 -> Pelvis to COM Position [m m m]/1
  body frame1/1 -> Pelvis to COM Velocity [m/s m/s m/s]/1
  PositionUsingRobotGeometry/7(lateral_com_position) -> Mux9/1
  "[z dz]"/1 -> "Vertical COM [m, m/s]"/1
  Switch/1 -> "[x dx]"/1, "[y dy]"/1, "[z dz]"/1, "[ddx, ddy, ddz]"/1
  "[y dy]"/1 -> "Lateral COM [m, m/s]"/1
  Demux/3 -> Kalman Filtering/5(GRFz [N])
  Demux/2 -> Kalman Filtering/4(GRFy [N])
  Kalman Filtering/1("[x, dx, ddx] [m/s, m/s^2]") -> Mux5/1, Demux4/1
  Kalman Filtering/3("[z, dz, ddz] [m, m/s, m/s^2]") -> Demux1/1, Mux5/3
  Kalman Filtering/2("[y, dy, ddy] [m/s, m/s^2]") -> Demux6/1, Mux5/2
  Kalman Filtering/5("[y, dy, ddy] uncertainty") -> Mux1/2
  Kalman Filtering/4("[x, dx, ddx] uncertainty") -> Mux1/1
  Kalman Filtering/6("[z, dz, ddz] uncertainty") -> Mux1/3
  PositionUsingRobotGeometry/9(vertical_com_position) -> Mux/1
  PositionUsingRobotGeometry/10(vertical_com_velocity) -> Mux/2
  Mux/1 -> Mux3/3, Demux3/1, Kalman Filtering/10("Initial [z, dz, ddz] [m m/s m/s^2]")
  PositionUsingRobotGeometry/8(lateral_com_velocity) -> Mux9/2
  PositionUsingRobotGeometry/6(horizontal_com_velocity) -> Mux8/2
  [RightLeftPrimary] -> Switch2/2
  Mux17/1 -> Switch2/3
  Mux16/1 -> Switch2/1
  Switch2/1 -> Demux11/1
  Demux11/2 -> Foot to COM Velocity [m/s m/s m/s]/1
  Demux11/1 -> Foot to COM Position [m m m]/1
  body frame2/1 -> Mux17/1
  body frame3/1 -> Mux17/2
  body frame5/1 -> Mux16/2
  body frame4/1 -> Mux16/1
  Flight [1/0]/1 -> Detect Decrease/1
  Detect Decrease/1 -> Kalman Filtering/12(Entering Stance [1/0])
  Mux4/1 -> Z Kalman Output/3
  Mux6/1 -> Z Kalman Output/1
  Demux1/2 -> Mux10/2
  Demux1/1 -> Mux6/2
  Mux10/1 -> Z Kalman Output/2
  Demux1/3 -> Mux4/2
  Demux3/1 -> Mux6/1
  Demux3/2 -> Mux10/1
  Demux3/3 -> Mux4/1
  Mux15/1 -> Y Kalman Output/3
  Mux18/1 -> Y Kalman Output/1
  Demux6/2 -> Mux14/2
  Demux6/1 -> Mux18/2
  Mux14/1 -> Y Kalman Output/2
  Demux6/3 -> Mux15/2
  Demux7/1 -> Mux18/1
  Demux7/2 -> Mux14/1
  Demux7/3 -> Mux15/1
  ComputeKneePositions/1(front_knee_to_right_foot) -> Mux2/1
  ComputeKneePositions/2(back_knee_to_right_foot) -> Mux2/2
  ComputeKneePositions/3(front_knee_to_left_foot) -> L Front Back Knee to Foot/1, Mux7/1
  ComputeKneePositions/4(back_knee_to_left_foot) -> L Front Back Knee to Foot/2, Mux7/2
  Mux2/1 -> Right Knees to Foot [m m m] x2/1
  Mux7/1 -> Left Knees to Foot [m m m] x2/1
  Left Front [rad rad/s]/1 -> ComputeKneePositions/13(left_front_angle)
  Right Front [rad rad/s]/1 -> ComputeKneePositions/12(right_front_angle)
  Left Back [rad rad/s]/1 -> ComputeKneePositions/11(left_back_angle)
  Right Back [rad rad/s]/1 -> ComputeKneePositions/10(right_back_angle)
  [EnableKalmanFiltering] -> Switch/2
  PositionUsingRobotGeometry/1(com_left_foot) -> body frame6/1, body frame2/1, Kalman Filtering/1("COM from Left Foot [body, yawed, global]")
  PositionUsingRobotGeometry/2(dcom_left_foot) -> body frame7/1, body frame3/1
  PositionUsingRobotGeometry/3(com_right_foot) -> body frame8/1, body frame4/1, Kalman Filtering/2("COM from Right Foot [body, yawed, global]")
  PositionUsingRobotGeometry/4(dcom_right_foot) -> body frame9/1, body frame5/1
  [RightLeftPrimary] -> Switch1/2
  Mux20/1 -> Switch1/3
  Mux19/1 -> Switch1/1
  Switch1/1 -> Demux8/1
  Demux8/2 -> COM Velocity World [m/s m/s m/s]/1
  Demux8/1 -> COM Position World [m m m]/1
  body frame6/1 -> Mux20/1
  body frame7/1 -> Mux20/2
  body frame9/1 -> Mux19/2
  body frame8/1 -> Mux19/1
  Discrete Derivative1/1 -> Mux11/4

== system playback_data/Control/Actuator Control with Torque SEA commands/Contact Velocities/Velocity on Contact ==
  in : Inport
  Trigger : TriggerPort  ShowOutputPort=on  PortDimensions=1
  Subsystem : Subsystem
  out : Outport
  wires:
  Trigger/1 -> Subsystem/Enable
  Subsystem/1(out) -> out/1
  in/1 -> Subsystem/1(in)

== system playback_data/Control/Actuator Control with Torque SEA commands/Contact Velocities/Velocity on Contact1 ==
  in : Inport
  Trigger : TriggerPort  ShowOutputPort=on  PortDimensions=1
  Subsystem : Subsystem
  out : Outport
  wires:
  in/1 -> Subsystem/1(in)
  Subsystem/1(out) -> out/1
  Trigger/1 -> Subsystem/Enable

== system playback_data/Control/Actuator Control with Torque SEA commands/Contact Velocities/Velocity on Contact2 ==
  in : Inport
  Trigger : TriggerPort  ShowOutputPort=on  PortDimensions=1
  Subsystem : Subsystem
  out : Outport
  wires:
  in/1 -> Subsystem/1(in)
  Subsystem/1(out) -> out/1
  Trigger/1 -> Subsystem/Enable

== system playback_data/Control/Actuator Control with Torque SEA commands/Contact Velocities/Velocity on Contact3 ==
  in : Inport
  Trigger : TriggerPort  ShowOutputPort=on  PortDimensions=1
  Subsystem : Subsystem
  out : Outport
  wires:
  Trigger/1 -> Subsystem/Enable
  Subsystem/1(out) -> out/1
  in/1 -> Subsystem/1(in)

== system playback_data/Control/Actuator Control with Torque SEA commands/SEA Controller (Torque)/Antiresonance Compensation ==
  Torque : Inport
  Notch Filter (Flight) : DiscreteTransferFcn  Numerator=[K_notch_f1 K_notch_f1*A1_notch_f1 K_notch_f1*A2_notch_f1]  Denominator=[1 B1_notch_f1 B2_notch_f1]  SampleTime=sample_time
  Filtered Torque : Outport
  wires:
  Notch Filter (Flight)/1 -> Filtered Torque/1
  Torque/1 -> Notch Filter (Flight)/1

== system playback_data/Control/Actuator Control with Torque SEA commands/SEA Controller (Torque)/Friction Compensation ==
  Motor Velocity [rad/s] : Inport
  Gain2 : Gain  Gain=sea_coulomb_friction_direction_switch_sensitivity
  KdGain2 : Gain  Description=xPCTag(1)=kd_sea_torque;  Gain=sea_coulomb_friction
  Trigonometric Function : Trigonometry  Operator=tanh
  Friction Compensation [Nm] : Outport
  wires:
  Trigonometric Function/1 -> KdGain2/1
  Gain2/1 -> Trigonometric Function/1
  Motor Velocity [rad/s]/1 -> Gain2/1
  KdGain2/1 -> Friction Compensation [Nm]/1

== system playback_data/Control/Actuator Control with Torque SEA commands/SEA Controller (Torque)/Loaded Unloaded Switch ==
  Loaded Signal : Inport
  Unloaded Signal : Inport  Port=2
  Loaded/Unloaded [1/0] x4 : Inport  Port=3
  Demux : Demux
  Demux1 : Demux
  Demux2 : Demux
  Mux : Mux
  Switch{,1..3} (4 alike) : Switch  Criteria=u2 ~= 0
  Signal : Outport
  wires:
  Demux2/1 -> Switch/3
  Demux2/2 -> Switch1/3
  Demux2/3 -> Switch2/3
  Demux2/4 -> Switch3/3
  Unloaded Signal/1 -> Demux2/1
  Demux1/4 -> Switch3/1
  Demux1/3 -> Switch2/1
  Demux1/2 -> Switch1/1
  Demux1/1 -> Switch/1
  Loaded Signal/1 -> Demux1/1
  Demux/1 -> Switch/2
  Switch/1 -> Mux/1
  Mux/1 -> Signal/1
  Loaded/Unloaded [1/0] x4/1 -> Demux/1
  Switch3/1 -> Mux/4
  Switch2/1 -> Mux/3
  Switch1/1 -> Mux/2
  Demux/2 -> Switch1/2
  Demux/3 -> Switch2/2
  Demux/4 -> Switch3/2

== system playback_data/Control/Actuator Control with Torque SEA commands/SEA Controller (Torque)/critical damping ==
  p gain : Inport
  Gain : Gain  Gain=0.75
  Gain1 : Gain  Gain=2
  Gain2 : Gain  Gain=j_motor
  Spring Stiffness1 : Gain  Gain=1./k_sea_low
  Sqrt : Sqrt  SaturateOnIntegerOverflow=on
  d gain : Outport
  wires:
  p gain/1 -> Spring Stiffness1/1
  Gain/1 -> Gain1/1
  Sqrt/1 -> Gain/1
  Gain2/1 -> Sqrt/1
  Spring Stiffness1/1 -> Gain2/1
  Gain1/1 -> d gain/1

== system playback_data/Control/Actuator Control with Torque SEA commands/SEA Controller (Velocity)/Integrator ==
  Signal : Inport
  Reset [1/0] : Inport  Port=2
  Demux : Demux
  Demux1 : Demux
  Discrete-Time Integrator{,1..3} (4 alike) : DiscreteIntegrator  ExternalReset=rising  InitialConditionSetting=State (most efficient)  SampleTime=sample_time  LimitOutput=on  UpperSaturationLimit=1  LowerSaturationLimit=-1
  Mux : Mux
  Integrated : Outport
  wires:
  Signal/1 -> Demux/1
  Discrete-Time Integrator/1 -> Mux/1
  Reset [1/0]/1 -> Demux1/1
  Mux/1 -> Integrated/1
  Discrete-Time Integrator1/1 -> Mux/2
  Discrete-Time Integrator2/1 -> Mux/3
  Discrete-Time Integrator3/1 -> Mux/4
  Demux1/4 -> Discrete-Time Integrator3/2
  Demux1/3 -> Discrete-Time Integrator2/2
  Demux1/2 -> Discrete-Time Integrator1/2
  Demux1/1 -> Discrete-Time Integrator/2
  Demux/1 -> Discrete-Time Integrator/1
  Demux/2 -> Discrete-Time Integrator1/1
  Demux/3 -> Discrete-Time Integrator2/1
  Demux/4 -> Discrete-Time Integrator3/1
